simulink model "Lab_7"  (R2016a)
settings: Solver=VariableStepAuto  StartTime=0.0  StopTime=10.0  RelTol=1e-3
libraries: dspfdesign x1
settings Model: Creator=Student  LastModifiedBy=Student

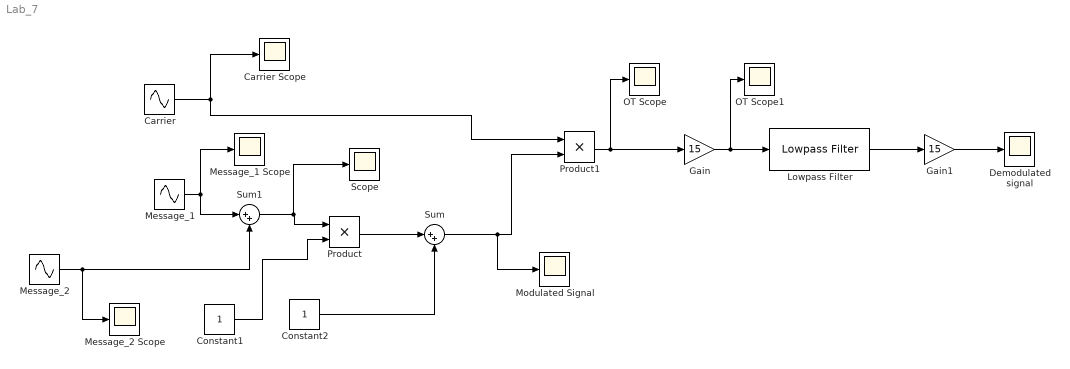
== system Lab_7 ==
  Carrier : Sin  Frequency=2*pi*50  SampleTime=1/5000
  "Carrier Scope " : Scope
  Constant1 : Constant  SampleTime=1/5000
  Constant2 : Constant  SampleTime=1/5000
  "Demodulated signal " : Scope
  Gain : Gain  Gain=15
  Gain1 : Gain  Gain=15
  Lowpass Filter : dspfdesign/Lowpass Filter  FilterType=FIR  DesignForMinimumOrder=on  FilterOrder=50  PassbandFrequency=8e3  StopbandFrequency=12e3  PassbandRipple=0.1  StopbandAttenuation=80  InheritSampleRate=off  SampleRate=44100  roundingMode=Floor  coeffsDataTypeStr=fixdt(1,16)  SimulateUsing=Interpreted execution
  "Message_1 " : Sin  Amplitude=2  Frequency=2*pi*4  SampleTime=1/5000
  "Message_1 Scope " : Scope
  Message_2 : Sin  Amplitude=3  Frequency=2*pi*6  SampleTime=1/5000
  Message_2 Scope : Scope
  Modulated Signal : Scope
  OT Scope : Scope
  OT Scope1 : Scope
  Product : Product
  Product1 : Product
  Scope : Scope
  Sum : Sum  Inputs=|++
  Sum1 : Sum  Inputs=|++
  wires:
  "Message_1 "/1 -> Sum1/1, "Message_1 Scope "/1
  Carrier/1 -> "Carrier Scope "/1, Product1/1
  Product1/1 -> Gain/1, OT Scope/1
  Product/1 -> Sum/1
  Constant2/1 -> Sum/2
  Sum/1 -> Modulated Signal/1, Product1/2
  Message_2/1 -> Sum1/2, Message_2 Scope/1
  Lowpass Filter/1 -> Gain1/1
  Gain1/1 -> "Demodulated signal "/1
  Gain/1 -> OT Scope1/1, Lowpass Filter/1
  Constant1/1 -> Product/2
  Sum1/1 -> Scope/1, Product/1
